simulink model "Simulink_Reis_4x4"  (R2021a)
settings: Solver=ode45  StartTime=0.0  StopTime=1000  RelTol=1e-3
model workspace (MAT data in the model file):
  Gm = tf
  Gm.IOSize_ = [2 2]
  Gm.Data_ = ltipack.tfdata
  Gm.Data_.num = {[0 87.8], [0 -86.4]; [0 108.2], [0 -109.6]}
  Gm.Data_.den = {[75 1], [75 1]; [75 1], [75 1]}
  Gm.Data_.Delay.Input = [0; 0]
  Gm.Data_.Delay.Output = [0; 0]
  Gm.Data_.Delay.IO = [0  0; 0  0]
  Gm.Data_.Ts = 0
undefined symbols (not defined in the file or in its folder): D, Did, Gfinal, kd_1, kd_2, kd_3, kd_4, ki_1, ki_2, ki_3, ki_4, kp_1, kp_2, kp_3, kp_4, Tdio
libraries: cstextras x18, pid_lib x4
Description:
  | The LTISystemBlockMIMO model shows how to use an LTI System block to represent a MIMO plant in a control system.
settings Model: Creator=The MathWorks, Inc.  LastModifiedBy=Grazielle
settings SolverCC: AlgebraicLoopSolver=LineSearch
settings DataIOCC: ReturnWorkspaceOutputs=off
settings DebuggingCC: SFMachineParentedDataDiag=warning  ArithmeticOperatorsInVariantConditions=warning
settings SFSimCC: SimUseLocalCustomCode=off  CustomCodeUndefinedFunction=UseInterfaceOnly
settings RTWCC: RTWUseLocalCustomCode=off
settings CodeAppCC: StateflowObjectComments=on
settings ConfigComp: CovMetricSettings=dswe

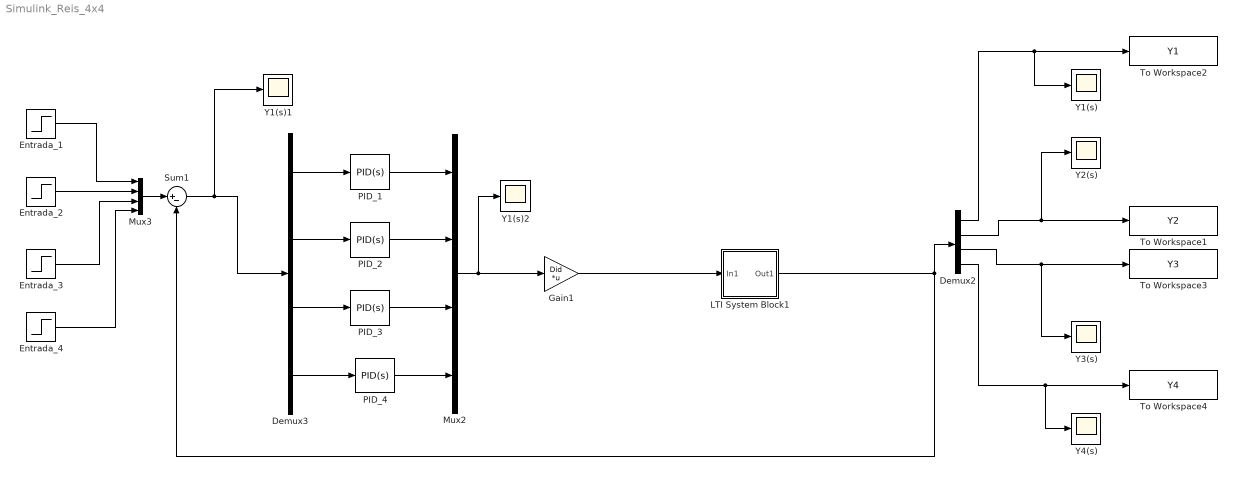
== system Simulink_Reis_4x4 ==
  Demux2 : Demux
  Demux3 : Demux
  Entrada_{1..4} (4 alike) : Step  SampleTime=0
  Gain1 : Gain  Gain=Did  Multiplication=Matrix(K*u)
  LTI System Block1 : Subsystem  AncestorBlock=cstblocks/LTI System  BlockChoice=CSS  mask(LTI Block){sys=Gfinal, IC=[]}
      mask prompts: sys "Control:simulink:LTIMaskLabel1"; IC "Control:simulink:LTIMaskLabel2"
      mask help: Control:simulink:LTIMaskDescription
      mask init:
      | try
      |    % read data to initialize mask variables
      |    [D,Ts,Tdi,Tdo,Tdio,x0,sysname]=...
      |       ltimask('Initialize',gcb,sys,IC);
      |    % update contents
      |    model = bdroot;
      |    df = get_param(model,'dirty');
      |    ltimask('UpdateDiagram',gcb,D,Ts,Tdio);
      |    try      
      |       % Attempt to modify locked library -> error
      |       % Makes block show ??? when loading CSTBLOCKS
      |       % for the first time
      |       set_param(model,'dirty',df)
      |    end
      | catch ME
      |    sys = [];  IC = [];   sysname = '???';
      |    throw(ME)
      | end
      mask Help: eval('ctrlguihelp(''ltisystemblock'');')
      mask Callback sys: ltimask('MaskLTICallback',gcb);
      mask DialogControl sys Prompt: LTI system variable
      mask DialogControl IC Prompt: Initial states (state-space only)
      mask Display: disp(sysname)
  Mux2 : Mux
  Mux3 : Mux
  PID_1 : pid_lib/PID Controller  Controller=PID  Form=Parallel  TimeDomain=Continuous-time  UseExternalTs=off  SampleTime=-1  IntegratorMethod=Forward Euler  FilterMethod=Forward Euler  ControllerParametersSource=internal  P=kp_1  I=ki_1  D=kd_1  UseFilter=on  N=0  TunerSelectOption=Transfer Function Based (PID Tuner App)  InitialConditionSource=internal  InitialConditionForIntegrator=0  InitialConditionForFilter=0  DifferentiatorICPrevScaledInput=0  ExternalReset=none  TrackingMode=off  Kt=1  LimitOutput=off  SatLimitsSource=internal  UpperSaturationLimit=inf  LowerSaturationLimit=-inf  LinearizeAsGain=on  AntiWindupMode=none  Kb=1  POutMin=[]  POutMax=[]  IOutMin=[]  IOutMax=[]  DOutMin=[]  DOutMax=[]  NOutMin=[]  NOutMax=[]  SumOutMin=[]  SumOutMax=[]  SaturationOutMin=[]  SaturationOutMax=[]  PParamMin=[]  PParamMax=[]  IParamMin=[]  IParamMax=[]  DParamMin=[]  DParamMax=[]  NParamMin=[]  NParamMax=[]  KbParamMin=[]  KbParamMax=[]  KtParamMin=[]  KtParamMax=[]  KbOutMin=[]  KbOutMax=[]  KtOutMin=[]  KtOutMax=[]  IntegratorOutMin=[]  IntegratorOutMax=[]  FilterOutMin=[]  FilterOutMax=[]  SumI1OutMin=[]  SumI1OutMax=[]  SumI2OutMin=[]  SumI2OutMax=[]  SumI3OutMin=[]  SumI3OutMax=[]  SumI4OutMin=[]  SumI4OutMax=[]  SumDOutMin=[]  SumDOutMax=[]  DifferentiatorOutMin=[]  DifferentiatorOutMax=[]  FilterDiffOutCoefMin=[]  FilterDiffOutCoefMax=[]  ReciprocalOutMin=[]  ReciprocalOutMax=[]  SumDenOutMin=[]  SumDenOutMax=[]  SumNumOutMin=[]  SumNumOutMax=[]  DivideOutMin=[]  DivideOutMax=[]  UdiffTsProdOutMin=[]  UdiffTsProdOutMax=[]  NTsProdOutMin=[]  NTsProdOutMax=[]  UintegralTsProdOutMin=[]  UintegralTsProdOutMax=[]  UngainTsProdOutMin=[]  UngainTsProdOutMax=[]  IntegratorContinuousStateAttributes=''  IntegratorStateMustResolveToSignalObject=off  IntegratorRTWStateStorageClass=Auto  FilterContinuousStateAttributes=''  FilterStateMustResolveToSignalObject=off  FilterRTWStateStorageClass=Auto  ParallelPVariant=InternalParameters  IdealPVariant=Disabled  IVariant=InternalParameters  DVariant=InternalParameters  IntegratorVariant=Continuous  SatVariant=Disabled  AWVariant=Passthrough  PCopyVariant=Disabled  TRVariant=Disabled  FdbkBlocksVariant=Forward  IdealPFdbkVariant=Disabled  SatFdbkVariant=Disabled  DerivativeFilterVariant=ContFilter  NVariant=InternalParameters  NCopyVariant=Disabled  FilterICVariant=InternalICsFilter  IntegratorICVariant=InternalICs  ExternalResetVariant=Disabled  TRSumVariant=Passthrough  SumFdbkVariant=Disabled  SumVariant=Sum_PID  TsampFilterVariant=InternalTs  TsampNgainVariant=Passthrough  TsampIntegralVariant=Passthrough  ExternalSaturationOutDataTypeStr=Inherit: Same as second input
  PID_2 : pid_lib/PID Controller  Controller=PID  Form=Parallel  TimeDomain=Continuous-time  UseExternalTs=off  SampleTime=-1  IntegratorMethod=Forward Euler  FilterMethod=Forward Euler  ControllerParametersSource=internal  P=kp_2  I=ki_2  D=kd_2  UseFilter=on  N=0  TunerSelectOption=Transfer Function Based (PID Tuner App)  InitialConditionSource=internal  InitialConditionForIntegrator=0  InitialConditionForFilter=0  DifferentiatorICPrevScaledInput=0  ExternalReset=none  TrackingMode=off  Kt=1  LimitOutput=off  SatLimitsSource=internal  UpperSaturationLimit=inf  LowerSaturationLimit=-inf  LinearizeAsGain=on  AntiWindupMode=none  Kb=1  POutMin=[]  POutMax=[]  IOutMin=[]  IOutMax=[]  DOutMin=[]  DOutMax=[]  NOutMin=[]  NOutMax=[]  SumOutMin=[]  SumOutMax=[]  SaturationOutMin=[]  SaturationOutMax=[]  PParamMin=[]  PParamMax=[]  IParamMin=[]  IParamMax=[]  DParamMin=[]  DParamMax=[]  NParamMin=[]  NParamMax=[]  KbParamMin=[]  KbParamMax=[]  KtParamMin=[]  KtParamMax=[]  KbOutMin=[]  KbOutMax=[]  KtOutMin=[]  KtOutMax=[]  IntegratorOutMin=[]  IntegratorOutMax=[]  FilterOutMin=[]  FilterOutMax=[]  SumI1OutMin=[]  SumI1OutMax=[]  SumI2OutMin=[]  SumI2OutMax=[]  SumI3OutMin=[]  SumI3OutMax=[]  SumI4OutMin=[]  SumI4OutMax=[]  SumDOutMin=[]  SumDOutMax=[]  DifferentiatorOutMin=[]  DifferentiatorOutMax=[]  FilterDiffOutCoefMin=[]  FilterDiffOutCoefMax=[]  ReciprocalOutMin=[]  ReciprocalOutMax=[]  SumDenOutMin=[]  SumDenOutMax=[]  SumNumOutMin=[]  SumNumOutMax=[]  DivideOutMin=[]  DivideOutMax=[]  UdiffTsProdOutMin=[]  UdiffTsProdOutMax=[]  NTsProdOutMin=[]  NTsProdOutMax=[]  UintegralTsProdOutMin=[]  UintegralTsProdOutMax=[]  UngainTsProdOutMin=[]  UngainTsProdOutMax=[]  IntegratorContinuousStateAttributes=''  IntegratorStateMustResolveToSignalObject=off  IntegratorRTWStateStorageClass=Auto  FilterContinuousStateAttributes=''  FilterStateMustResolveToSignalObject=off  FilterRTWStateStorageClass=Auto  ParallelPVariant=InternalParameters  IdealPVariant=Disabled  IVariant=InternalParameters  DVariant=InternalParameters  IntegratorVariant=Continuous  SatVariant=Disabled  AWVariant=Passthrough  PCopyVariant=Disabled  TRVariant=Disabled  FdbkBlocksVariant=Forward  IdealPFdbkVariant=Disabled  SatFdbkVariant=Disabled  DerivativeFilterVariant=ContFilter  NVariant=InternalParameters  NCopyVariant=Disabled  FilterICVariant=InternalICsFilter  IntegratorICVariant=InternalICs  ExternalResetVariant=Disabled  TRSumVariant=Passthrough  SumFdbkVariant=Disabled  SumVariant=Sum_PID  TsampFilterVariant=InternalTs  TsampNgainVariant=Passthrough  TsampIntegralVariant=Passthrough  ExternalSaturationOutDataTypeStr=Inherit: Same as second input
  PID_3 : pid_lib/PID Controller  Controller=PID  Form=Parallel  TimeDomain=Continuous-time  UseExternalTs=off  SampleTime=-1  IntegratorMethod=Forward Euler  FilterMethod=Forward Euler  ControllerParametersSource=internal  P=kp_3  I=ki_3  D=kd_3  UseFilter=on  N=0  TunerSelectOption=Transfer Function Based (PID Tuner App)  InitialConditionSource=internal  InitialConditionForIntegrator=0  InitialConditionForFilter=0  DifferentiatorICPrevScaledInput=0  ExternalReset=none  TrackingMode=off  Kt=1  LimitOutput=off  SatLimitsSource=internal  UpperSaturationLimit=inf  LowerSaturationLimit=-inf  LinearizeAsGain=on  AntiWindupMode=none  Kb=1  POutMin=[]  POutMax=[]  IOutMin=[]  IOutMax=[]  DOutMin=[]  DOutMax=[]  NOutMin=[]  NOutMax=[]  SumOutMin=[]  SumOutMax=[]  SaturationOutMin=[]  SaturationOutMax=[]  PParamMin=[]  PParamMax=[]  IParamMin=[]  IParamMax=[]  DParamMin=[]  DParamMax=[]  NParamMin=[]  NParamMax=[]  KbParamMin=[]  KbParamMax=[]  KtParamMin=[]  KtParamMax=[]  KbOutMin=[]  KbOutMax=[]  KtOutMin=[]  KtOutMax=[]  IntegratorOutMin=[]  IntegratorOutMax=[]  FilterOutMin=[]  FilterOutMax=[]  SumI1OutMin=[]  SumI1OutMax=[]  SumI2OutMin=[]  SumI2OutMax=[]  SumI3OutMin=[]  SumI3OutMax=[]  SumI4OutMin=[]  SumI4OutMax=[]  SumDOutMin=[]  SumDOutMax=[]  DifferentiatorOutMin=[]  DifferentiatorOutMax=[]  FilterDiffOutCoefMin=[]  FilterDiffOutCoefMax=[]  ReciprocalOutMin=[]  ReciprocalOutMax=[]  SumDenOutMin=[]  SumDenOutMax=[]  SumNumOutMin=[]  SumNumOutMax=[]  DivideOutMin=[]  DivideOutMax=[]  UdiffTsProdOutMin=[]  UdiffTsProdOutMax=[]  NTsProdOutMin=[]  NTsProdOutMax=[]  UintegralTsProdOutMin=[]  UintegralTsProdOutMax=[]  UngainTsProdOutMin=[]  UngainTsProdOutMax=[]  IntegratorContinuousStateAttributes=''  IntegratorStateMustResolveToSignalObject=off  IntegratorRTWStateStorageClass=Auto  FilterContinuousStateAttributes=''  FilterStateMustResolveToSignalObject=off  FilterRTWStateStorageClass=Auto  ParallelPVariant=InternalParameters  IdealPVariant=Disabled  IVariant=InternalParameters  DVariant=InternalParameters  IntegratorVariant=Continuous  SatVariant=Disabled  AWVariant=Passthrough  PCopyVariant=Disabled  TRVariant=Disabled  FdbkBlocksVariant=Forward  IdealPFdbkVariant=Disabled  SatFdbkVariant=Disabled  DerivativeFilterVariant=ContFilter  NVariant=InternalParameters  NCopyVariant=Disabled  FilterICVariant=InternalICsFilter  IntegratorICVariant=InternalICs  ExternalResetVariant=Disabled  TRSumVariant=Passthrough  SumFdbkVariant=Disabled  SumVariant=Sum_PID  TsampFilterVariant=InternalTs  TsampNgainVariant=Passthrough  TsampIntegralVariant=Passthrough  ExternalSaturationOutDataTypeStr=Inherit: Same as second input
  PID_4 : pid_lib/PID Controller  Controller=PID  Form=Parallel  TimeDomain=Continuous-time  UseExternalTs=off  SampleTime=-1  IntegratorMethod=Forward Euler  FilterMethod=Forward Euler  ControllerParametersSource=internal  P=kp_4  I=ki_4  D=kd_4  UseFilter=on  N=0  TunerSelectOption=Transfer Function Based (PID Tuner App)  InitialConditionSource=internal  InitialConditionForIntegrator=0  InitialConditionForFilter=0  DifferentiatorICPrevScaledInput=0  ExternalReset=none  TrackingMode=off  Kt=1  LimitOutput=off  SatLimitsSource=internal  UpperSaturationLimit=inf  LowerSaturationLimit=-inf  LinearizeAsGain=on  AntiWindupMode=none  Kb=1  POutMin=[]  POutMax=[]  IOutMin=[]  IOutMax=[]  DOutMin=[]  DOutMax=[]  NOutMin=[]  NOutMax=[]  SumOutMin=[]  SumOutMax=[]  SaturationOutMin=[]  SaturationOutMax=[]  PParamMin=[]  PParamMax=[]  IParamMin=[]  IParamMax=[]  DParamMin=[]  DParamMax=[]  NParamMin=[]  NParamMax=[]  KbParamMin=[]  KbParamMax=[]  KtParamMin=[]  KtParamMax=[]  KbOutMin=[]  KbOutMax=[]  KtOutMin=[]  KtOutMax=[]  IntegratorOutMin=[]  IntegratorOutMax=[]  FilterOutMin=[]  FilterOutMax=[]  SumI1OutMin=[]  SumI1OutMax=[]  SumI2OutMin=[]  SumI2OutMax=[]  SumI3OutMin=[]  SumI3OutMax=[]  SumI4OutMin=[]  SumI4OutMax=[]  SumDOutMin=[]  SumDOutMax=[]  DifferentiatorOutMin=[]  DifferentiatorOutMax=[]  FilterDiffOutCoefMin=[]  FilterDiffOutCoefMax=[]  ReciprocalOutMin=[]  ReciprocalOutMax=[]  SumDenOutMin=[]  SumDenOutMax=[]  SumNumOutMin=[]  SumNumOutMax=[]  DivideOutMin=[]  DivideOutMax=[]  UdiffTsProdOutMin=[]  UdiffTsProdOutMax=[]  NTsProdOutMin=[]  NTsProdOutMax=[]  UintegralTsProdOutMin=[]  UintegralTsProdOutMax=[]  UngainTsProdOutMin=[]  UngainTsProdOutMax=[]  IntegratorContinuousStateAttributes=''  IntegratorStateMustResolveToSignalObject=off  IntegratorRTWStateStorageClass=Auto  FilterContinuousStateAttributes=''  FilterStateMustResolveToSignalObject=off  FilterRTWStateStorageClass=Auto  ParallelPVariant=InternalParameters  IdealPVariant=Disabled  IVariant=InternalParameters  DVariant=InternalParameters  IntegratorVariant=Continuous  SatVariant=Disabled  AWVariant=Passthrough  PCopyVariant=Disabled  TRVariant=Disabled  FdbkBlocksVariant=Forward  IdealPFdbkVariant=Disabled  SatFdbkVariant=Disabled  DerivativeFilterVariant=ContFilter  NVariant=InternalParameters  NCopyVariant=Disabled  FilterICVariant=InternalICsFilter  IntegratorICVariant=InternalICs  ExternalResetVariant=Disabled  TRSumVariant=Passthrough  SumFdbkVariant=Disabled  SumVariant=Sum_PID  TsampFilterVariant=InternalTs  TsampNgainVariant=Passthrough  TsampIntegralVariant=Passthrough  ExternalSaturationOutDataTypeStr=Inherit: Same as second input
  Sum1 : Sum  Inputs=|+-
  To Workspace1 : ToWorkspace  VariableName=Y2  SaveFormat=Timeseries  SampleTime=-1
  To Workspace2 : ToWorkspace  VariableName=Y1  SaveFormat=Timeseries  SampleTime=-1
  To Workspace3 : ToWorkspace  VariableName=Y3  SaveFormat=Timeseries  SampleTime=-1
  To Workspace4 : ToWorkspace  VariableName=Y4  SaveFormat=Timeseries  SampleTime=-1
  Y1(s) : Scope
  Y1(s)1 : Scope
  Y1(s)2 : Scope
  Y2(s) : Scope
  Y3(s) : Scope
  Y4(s) : Scope
  wires:
  Entrada_1/1 -> Mux3/1
  Sum1/1 -> Y1(s)1/1, Demux3/1
  Mux2/1 -> Y1(s)2/1, Gain1/1
  Gain1/1 -> LTI System Block1/1(In1)
  Mux3/1 -> Sum1/1
  Entrada_2/1 -> Mux3/2
  Demux3/3 -> PID_3/1
  PID_3/1 -> Mux2/3
  Demux3/4 -> PID_4/1
  PID_4/1 -> Mux2/4
  Demux3/2 -> PID_2/1
  PID_2/1 -> Mux2/2
  Demux3/1 -> PID_1/1
  PID_1/1 -> Mux2/1
  Entrada_3/1 -> Mux3/3
  Entrada_4/1 -> Mux3/4
  Demux2/1 -> Y1(s)/1, To Workspace2/1
  Demux2/2 -> Y2(s)/1, To Workspace1/1
  LTI System Block1/1(Out1) -> Sum1/2, Demux2/1
  Demux2/3 -> Y3(s)/1, To Workspace3/1
  Demux2/4 -> Y4(s)/1, To Workspace4/1

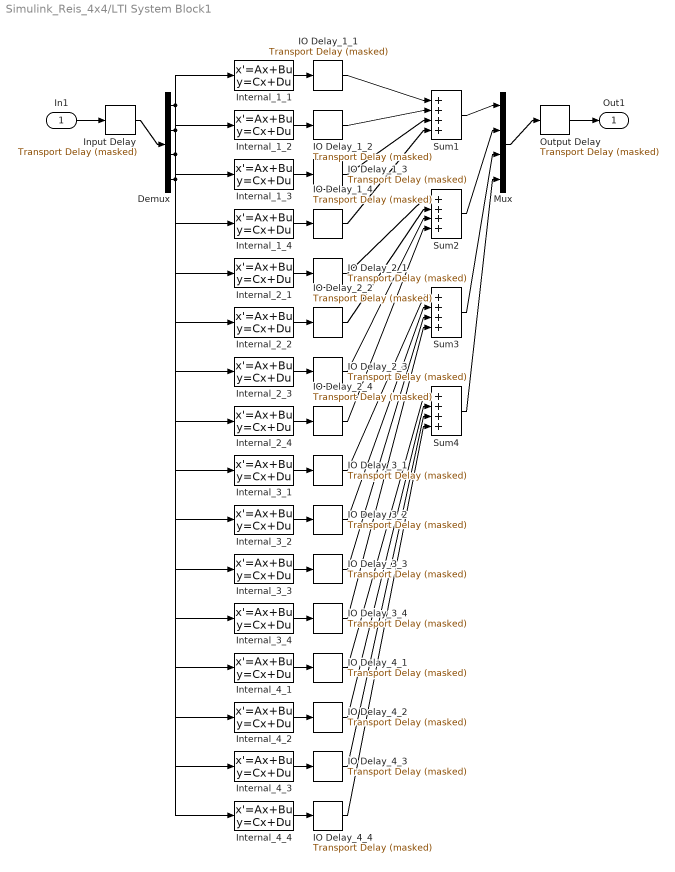
== system Simulink_Reis_4x4/LTI System Block1 ==
  In1 : Inport
  Demux : Demux
  IO Delay_1_1 : cstextras/Transport Delay (masked)  Td=Tdio(1,1)  u0=0  bufsize=1024
      settings: SourceProductBaseCode=CT
  IO Delay_1_2 : cstextras/Transport Delay (masked)  Td=Tdio(1,2)  u0=0  bufsize=1024
      settings: SourceProductBaseCode=CT
  IO Delay_1_3 : cstextras/Transport Delay (masked)  Td=Tdio(1,3)  u0=0  bufsize=1024
      settings: SourceProductBaseCode=CT
  IO Delay_1_4 : cstextras/Transport Delay (masked)  Td=Tdio(1,4)  u0=0  bufsize=1024
      settings: SourceProductBaseCode=CT
  IO Delay_2_1 : cstextras/Transport Delay (masked)  Td=Tdio(2,1)  u0=0  bufsize=1024
      settings: SourceProductBaseCode=CT
  IO Delay_2_2 : cstextras/Transport Delay (masked)  Td=Tdio(2,2)  u0=0  bufsize=1024
      settings: SourceProductBaseCode=CT
  IO Delay_2_3 : cstextras/Transport Delay (masked)  Td=Tdio(2,3)  u0=0  bufsize=1024
      settings: SourceProductBaseCode=CT
  IO Delay_2_4 : cstextras/Transport Delay (masked)  Td=Tdio(2,4)  u0=0  bufsize=1024
      settings: SourceProductBaseCode=CT
  IO Delay_3_1 : cstextras/Transport Delay (masked)  Td=Tdio(3,1)  u0=0  bufsize=1024
      settings: SourceProductBaseCode=CT
  IO Delay_3_2 : cstextras/Transport Delay (masked)  Td=Tdio(3,2)  u0=0  bufsize=1024
      settings: SourceProductBaseCode=CT
  IO Delay_3_3 : cstextras/Transport Delay (masked)  Td=Tdio(3,3)  u0=0  bufsize=1024
      settings: SourceProductBaseCode=CT
  IO Delay_3_4 : cstextras/Transport Delay (masked)  Td=Tdio(3,4)  u0=0  bufsize=1024
      settings: SourceProductBaseCode=CT
  IO Delay_4_1 : cstextras/Transport Delay (masked)  Td=Tdio(4,1)  u0=0  bufsize=1024
      settings: SourceProductBaseCode=CT
  IO Delay_4_2 : cstextras/Transport Delay (masked)  Td=Tdio(4,2)  u0=0  bufsize=1024
      settings: SourceProductBaseCode=CT
  IO Delay_4_3 : cstextras/Transport Delay (masked)  Td=Tdio(4,3)  u0=0  bufsize=1024
      settings: SourceProductBaseCode=CT
  IO Delay_4_4 : cstextras/Transport Delay (masked)  Td=Tdio(4,4)  u0=0  bufsize=1024
      settings: SourceProductBaseCode=CT
  Input Delay : cstextras/Transport Delay (masked)  Td=Tdi  u0=0  bufsize=1024
      settings: SourceProductBaseCode=CT
  Internal_1_1 : StateSpace  A=D(1,1).a  B=D(1,1).b  C=D(1,1).c  D=D(1,1).d
  Internal_1_2 : StateSpace  A=D(1,2).a  B=D(1,2).b  C=D(1,2).c  D=D(1,2).d
  Internal_1_3 : StateSpace  A=D(1,3).a  B=D(1,3).b  C=D(1,3).c  D=D(1,3).d
  Internal_1_4 : StateSpace  A=D(1,4).a  B=D(1,4).b  C=D(1,4).c  D=D(1,4).d
  Internal_2_1 : StateSpace  A=D(2,1).a  B=D(2,1).b  C=D(2,1).c  D=D(2,1).d
  Internal_2_2 : StateSpace  A=D(2,2).a  B=D(2,2).b  C=D(2,2).c  D=D(2,2).d
  Internal_2_3 : StateSpace  A=D(2,3).a  B=D(2,3).b  C=D(2,3).c  D=D(2,3).d
  Internal_2_4 : StateSpace  A=D(2,4).a  B=D(2,4).b  C=D(2,4).c  D=D(2,4).d
  Internal_3_1 : StateSpace  A=D(3,1).a  B=D(3,1).b  C=D(3,1).c  D=D(3,1).d
  Internal_3_2 : StateSpace  A=D(3,2).a  B=D(3,2).b  C=D(3,2).c  D=D(3,2).d
  Internal_3_3 : StateSpace  A=D(3,3).a  B=D(3,3).b  C=D(3,3).c  D=D(3,3).d
  Internal_3_4 : StateSpace  A=D(3,4).a  B=D(3,4).b  C=D(3,4).c  D=D(3,4).d
  Internal_4_1 : StateSpace  A=D(4,1).a  B=D(4,1).b  C=D(4,1).c  D=D(4,1).d
  Internal_4_2 : StateSpace  A=D(4,2).a  B=D(4,2).b  C=D(4,2).c  D=D(4,2).d
  Internal_4_3 : StateSpace  A=D(4,3).a  B=D(4,3).b  C=D(4,3).c  D=D(4,3).d
  Internal_4_4 : StateSpace  A=D(4,4).a  B=D(4,4).b  C=D(4,4).c  D=D(4,4).d
  Mux : Mux
  Output Delay : cstextras/Transport Delay (masked)  Td=Tdo  u0=0  bufsize=1024
      settings: SourceProductBaseCode=CT
  Sum{1..4} (4 alike) : Sum  Inputs=++++
  Out1 : Outport  InitialOutput=0  VectorParamsAs1DForOutWhenUnconnected=off
  wires:
  In1/1 -> Input Delay/1
  Output Delay/1 -> Out1/1
  Input Delay/1 -> Demux/1
  Mux/1 -> Output Delay/1
  Sum1/1 -> Mux/1
  Sum2/1 -> Mux/2
  Sum3/1 -> Mux/3
  Sum4/1 -> Mux/4
  Demux/1 -> Internal_1_1/1, Internal_2_1/1, Internal_3_1/1, Internal_4_1/1
  Internal_1_1/1 -> IO Delay_1_1/1
  IO Delay_1_1/1 -> Sum1/1
  Demux/2 -> Internal_1_2/1, Internal_2_2/1, Internal_3_2/1, Internal_4_2/1
  Internal_1_2/1 -> IO Delay_1_2/1
  IO Delay_1_2/1 -> Sum1/2
  Demux/3 -> Internal_1_3/1, Internal_2_3/1, Internal_3_3/1, Internal_4_3/1
  Internal_1_3/1 -> IO Delay_1_3/1
  IO Delay_1_3/1 -> Sum1/3
  Demux/4 -> Internal_1_4/1, Internal_2_4/1, Internal_3_4/1, Internal_4_4/1
  Internal_1_4/1 -> IO Delay_1_4/1
  IO Delay_1_4/1 -> Sum1/4
  Internal_2_1/1 -> IO Delay_2_1/1
  IO Delay_2_1/1 -> Sum2/1
  Internal_2_2/1 -> IO Delay_2_2/1
  IO Delay_2_2/1 -> Sum2/2
  Internal_2_3/1 -> IO Delay_2_3/1
  IO Delay_2_3/1 -> Sum2/3
  Internal_2_4/1 -> IO Delay_2_4/1
  IO Delay_2_4/1 -> Sum2/4
  Internal_3_1/1 -> IO Delay_3_1/1
  IO Delay_3_1/1 -> Sum3/1
  Internal_3_2/1 -> IO Delay_3_2/1
  IO Delay_3_2/1 -> Sum3/2
  Internal_3_3/1 -> IO Delay_3_3/1
  IO Delay_3_3/1 -> Sum3/3
  Internal_3_4/1 -> IO Delay_3_4/1
  IO Delay_3_4/1 -> Sum3/4
  Internal_4_1/1 -> IO Delay_4_1/1
  IO Delay_4_1/1 -> Sum4/1
  Internal_4_2/1 -> IO Delay_4_2/1
  IO Delay_4_2/1 -> Sum4/2
  Internal_4_3/1 -> IO Delay_4_3/1
  IO Delay_4_3/1 -> Sum4/3
  Internal_4_4/1 -> IO Delay_4_4/1
  IO Delay_4_4/1 -> Sum4/4
